simulink model "SimuDemonstrateurMoteur"  (R2015a)
settings: Solver=ode45  StartTime=0.0  StopTime=10.0  RelTol=1e-3
values from neighbouring files (symbols this model uses):
  Cn = 3e-4    (= 0.0003)    [MoteurScript.m]
  J2 = TauM2*mu    (= 9.94897959184e-05)    [MoteurScript.m]
  Kc = 3.5/100    (= 0.035)    [MoteurScript.m]
  Ke = 3.6/1000*60/(2*pi)    (= 0.0343774677078)    [MoteurScript.m]
  Kg = 0.105    [MoteurScript.m]
  Kr = 1/9    (= 0.111111111111)    [MoteurScript.m]
  Ks = 10    [MoteurScript.m]
  L = 0.8e-3    (= 0.0008)    [MoteurScript.m]
  mu = J1/TauM1    (= 0.000198979591837)    [MoteurScript.m]
  R = 6.2    [MoteurScript.m]
  Rchn = 100    [MoteurScript.m]
  rCn = Cn/2    (= 0.00015)    [MoteurScript.m]
  rRch = 0.5    [MoteurScript.m]
settings Model: Creator=sylvain  LastModifiedBy=David
settings OptimizationCC: ExpressionDepthLimit=2147483647
settings DebuggingCC: UnderspecifiedInitializationDetection=Classic  MergeDetectMultiDrivingBlocksExec=none  SolverPrmCheckMsg=warning  StateNameClashWarn=warning

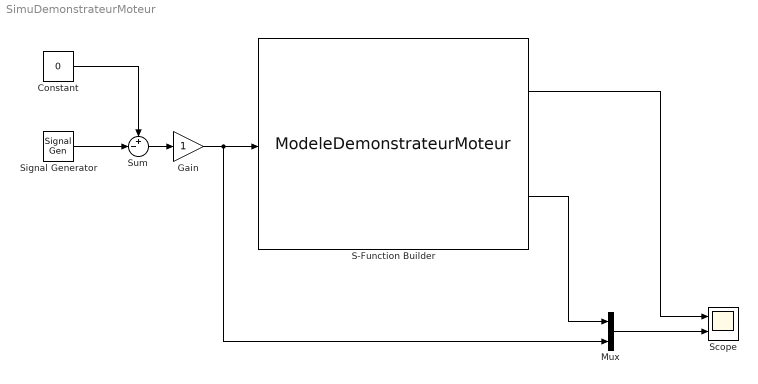
== system SimuDemonstrateurMoteur ==
  Constant : Constant  Value=0
  Gain : Gain
  Mux : Mux  Inputs=2
  S-Function Builder : S-Function  InitFcn=try, set_param(gcb,'FunctionName','ModeleDemonstrateurMoteur'), end  FunctionName=ModeleDemonstrateurMoteur  Parameters=R,L,Ke,Kc,mu,J2,Cn,rCn,2*rand(1)-1,Ks,Kr,Kg,0.01,Rchn,rRch,2*rand(1)-1  SFunctionModules=ModeleDemonstrateurMoteur_wrapper  mask(S-Function Builder){}
      mask help: Simulink:masks:SFunctionBuilder_MD
      mask init:
      | val = [[.9  0.75 0.75 1 1 .9 .9 1]',[1 1 0.75 0.75 .9 .9 1 .9]'];try , sys = get_param(gcb,'SfunBuilderFcnName');if isempty(sys), sys = get_param(gcb,'FunctionName'); end,catch, sys = get_param(gcb,'FunctionName'); end
      settings: CopyFcn=set_param(gcbh,'LinkStatus','none')  PreSaveFcn=try, set_param(gcb,'FunctionName','ModeleDemonstrateurMoteur'), end  OpenFcn=sfunctionwizard(gcbh)
      mask Display: plot(val(:,1),val(:,2)),disp(sys), port_label('input',1,'Vm'), port_label('output',1,'Vs'), port_label('output',2,'Vg')
  Scope : Scope  NumInputPorts=2
      settings: YMin=1.15~-0.7  YMax=1.675~0.7
  Signal Generator : SignalGenerator  WaveForm=square  Frequency=0.2
  Sum : Sum  Inputs=+-|
  wires:
  Signal Generator/1 -> Sum/2
  Constant/1 -> Sum/1
  Sum/1 -> Gain/1
  Gain/1 -> Mux/2, S-Function Builder/1
  S-Function Builder/2 -> Mux/1
  Mux/1 -> Scope/2
  S-Function Builder/1 -> Scope/1
